simulink model "MODELofpV1MODULE"  (R2023a)
settings: Solver=VariableStepAuto  StartTime=0.0  StopTime=2  RelTol=1e-3
libraries: spsPVArrayLib x6, spsDiodeLib x3, spsControlledVoltageSourceLib x1, spsCurrentMeasurementLib x1, simulink x1, spsVoltageMeasurementLib x1, sps_lib x1
settings Model: Creator=hp  LastModifiedBy=ask
settings SolverCC: AlgebraicLoopSolver=TrustRegion
settings DataIOCC: ReturnWorkspaceOutputs=off
settings DebuggingCC: UnconnectedInputMsg=warning  UnconnectedOutputMsg=warning  UnconnectedLineMsg=warning  ArithmeticOperatorsInVariantConditions=warning
settings ModelReferenceCC: EnableRefExpFcnMdlSchedulingChecks=on
settings SFSimCC: SimUseLocalCustomCode=off  CustomCodeUndefinedFunction=UseInterfaceOnly
settings RTWCC: RTWUseLocalCustomCode=off
settings CodeAppCC: StateflowObjectComments=on
settings SimscapeCC: SimscapeNormalizeSystem=off

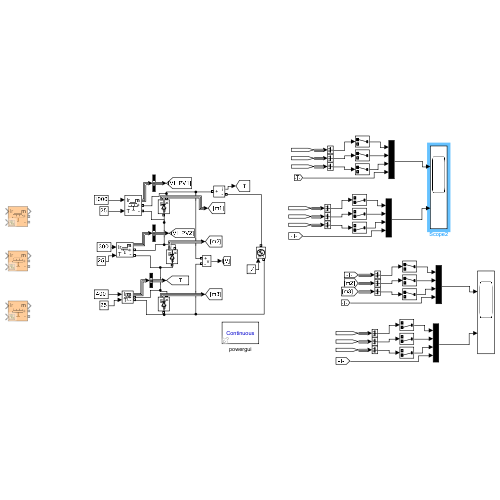
[thumbnail: Simulink's stored preview of the top-level diagram]
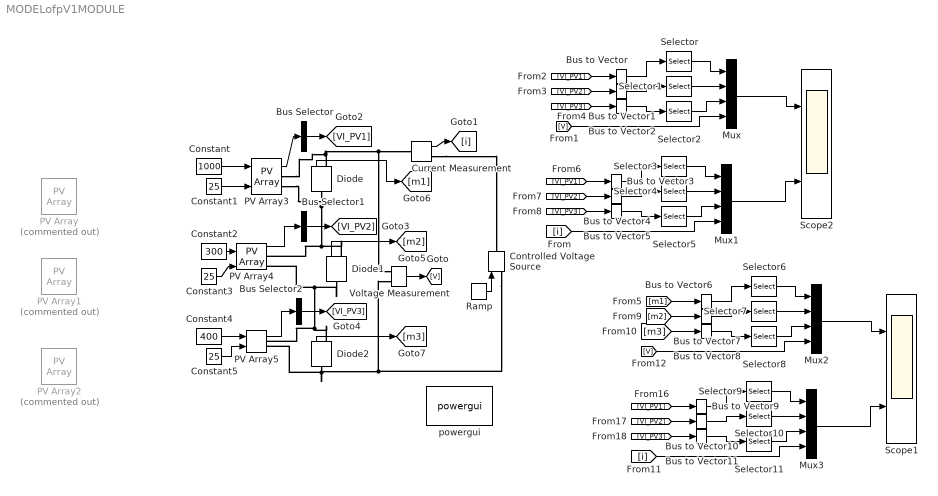
== system MODELofpV1MODULE ==
  Bus Selector : BusSelector  OutputSignals=V_PV,I_PV  OutputAsBus=on
  Bus Selector1 : BusSelector  OutputSignals=V_PV,I_PV  OutputAsBus=on
  Bus Selector2 : BusSelector  OutputSignals=V_PV,I_PV  OutputAsBus=on
  Bus to Vector{,1..11} (12 alike) : BusToVector
  Constant : Constant  Value=1000
  Constant1 : Constant  Value=25
  Constant2 : Constant  Value=300
  Constant3 : Constant  Value=25
  Constant4 : Constant  Value=400
  Constant5 : Constant  Value=25
  Controlled Voltage Source : spsControlledVoltageSourceLib/Controlled Voltage Source  Initialize=on  Source_Type=AC  Amplitude=0  Phase=0  Frequency=0  Measurements=None
  Current Measurement : spsCurrentMeasurementLib/Current Measurement  PhasorSimulation=off  OutputType=Complex  PSBequivalent=0
  Diode : spsDiodeLib/Diode  Ron=0.001  Lon=0  Vf=0.7  IC=0  UseSnubber=off  Rs=1e5*inf  Cs=inf  Measurements=on
  Diode1 : spsDiodeLib/Diode  Ron=0.001  Lon=0  Vf=0.7  IC=0  UseSnubber=off  Rs=1e5*inf  Cs=inf  Measurements=on
  Diode2 : spsDiodeLib/Diode  Ron=0.001  Lon=0  Vf=0.7  IC=0  UseSnubber=off  Rs=1e5*inf  Cs=inf  Measurements=on
  Mux{,1..3} (4 alike) : Mux
  PV Array : spsPVArrayLib/PV Array  Commented=on  Npar=1  Nser=1  PlotType=one module @ 25 deg.C & specified irradiances  S_vec="[ 1000  500  100 ]"  Temp_C_vec="[ 1000 500   ]"  ModuleName=User-defined  PlotWhenSelected=off  Pm=99.4224  Ncell=60/3  Voc=37.92*20/60  Isc=8.62  Vm=36.96*20/60  Im=8.07  beta_Voc_pc=-0.33969  alpha_Isc_pc=0.063701  beta_Voc=-0.042937  alpha_Isc=0.005491  IL=10.4557  I0=1.4325e-09  nI=1.3575  Rsh=1.8855  Rs=0.028506  RobustModel=off  RobustCellTemperature=313.3991  BAL=off  Tc=1e-6  Tfilter=5e-5
  PV Array1 : spsPVArrayLib/PV Array  Commented=on  Npar=1  Nser=1  PlotType=one module @ 25 deg.C & specified irradiances  S_vec="[ 1000  500  100 ]"  Temp_C_vec="[ 1000 500   ]"  ModuleName=User-defined  PlotWhenSelected=off  Pm=99.4224  Ncell=60/3  Voc=37.92*20/60  Isc=8.62  Vm=36.96*20/60  Im=8.07  beta_Voc_pc=-0.33969  alpha_Isc_pc=0.063701  beta_Voc=-0.042937  alpha_Isc=0.005491  IL=10.4557  I0=1.4325e-09  nI=1.3575  Rsh=1.8855  Rs=0.028506  RobustModel=off  RobustCellTemperature=313.3991  BAL=off  Tc=1e-6  Tfilter=5e-5
  PV Array2 : spsPVArrayLib/PV Array  Commented=on  Npar=1  Nser=1  PlotType=one module @ 25 deg.C & specified irradiances  S_vec="[ 1000  500  100 ]"  Temp_C_vec="[ 1000 500   ]"  ModuleName=User-defined  PlotWhenSelected=off  Pm=99.4224  Ncell=60/3  Voc=37.92*20/60  Isc=8.62  Vm=36.96*20/60  Im=8.07  beta_Voc_pc=-0.33969  alpha_Isc_pc=0.063701  beta_Voc=-0.042937  alpha_Isc=0.005491  IL=10.4557  I0=1.4325e-09  nI=1.3575  Rsh=1.8855  Rs=0.028506  RobustModel=off  RobustCellTemperature=313.3991  BAL=off  Tc=1e-6  Tfilter=5e-5
  PV Array3 : spsPVArrayLib/PV Array  Npar=1  Nser=1  PlotType=one module @ 25 deg.C & specified irradiances  S_vec="[ 1000  500  100 ]"  Temp_C_vec="[ 45 25  ]"  ModuleName=User-defined  PlotWhenSelected=off  Pm=99.4224  Ncell=60/3  Voc=37.92*20/60  Isc=8.62  Vm=36.96*20/60  Im=8.07  beta_Voc_pc=-0.36099  alpha_Isc_pc=0.063701  beta_Voc=-0.045629  alpha_Isc=0.005491  IL=10.5138  I0=5.8458e-10  nI=1.3056  Rsh=1.8742  Rs=0.043022  RobustModel=off  RobustCellTemperature=313.3991  BAL=on  Tc=1e-6  Tfilter=5e-5
  PV Array4 : spsPVArrayLib/PV Array  Npar=1  Nser=1  PlotType=one module @ 25 deg.C & specified irradiances  S_vec="[ 1000  500  100 ]"  Temp_C_vec="[ 45 25  ]"  ModuleName=User-defined  PlotWhenSelected=off  Pm=99.4224  Ncell=60/3  Voc=37.92*20/60  Isc=8.62  Vm=36.96*20/60  Im=8.07  beta_Voc_pc=-0.36099  alpha_Isc_pc=0.063701  beta_Voc=-0.045629  alpha_Isc=0.005491  IL=10.5138  I0=5.8458e-10  nI=1.3056  Rsh=1.8742  Rs=0.043022  RobustModel=off  RobustCellTemperature=313.3991  BAL=on  Tc=1e-6  Tfilter=5e-5
  PV Array5 : spsPVArrayLib/PV Array  Npar=1  Nser=1  PlotType=one module @ 25 deg.C & specified irradiances  S_vec="[ 1000  500  100 ]"  Temp_C_vec="[ 45 25  ]"  ModuleName=User-defined  PlotWhenSelected=off  Pm=99.4224  Ncell=60/3  Voc=37.92*20/60  Isc=8.62  Vm=36.96*20/60  Im=8.07  beta_Voc_pc=-0.36099  alpha_Isc_pc=0.063701  beta_Voc=-0.045629  alpha_Isc=0.005491  IL=10.5138  I0=5.8458e-10  nI=1.3056  Rsh=1.8742  Rs=0.043022  RobustModel=off  RobustCellTemperature=313.3991  BAL=on  Tc=1e-6  Tfilter=5e-5
  Ramp : simulink/Sources/Ramp  slope=37.92  start=0  InitialOutput=0
  Scope1 : Scope  NumInputPorts=2
  Scope2 : Scope  NumInputPorts=2
  Selector{,1..2,6..8} (6 alike) : Selector  InputPortWidth=2  IndexOptions=Index vector (dialog)  Indices=[1]  OutputSizes=1
  Selector{3..5,9..11} (6 alike) : Selector  InputPortWidth=2  IndexOptions=Index vector (dialog)  Indices=[2]  OutputSizes=1
  Voltage Measurement : spsVoltageMeasurementLib/Voltage Measurement  PhasorSimulation=off  OutputType=Complex  PSBequivalent=0
  powergui : sps_lib/powergui  Priority=1  SimulationMode=Continuous  SampleTime=50e-6  frequency=60  Iterations=50  frequencyindice=0  Pbase=100e6  ErrMax=1e-4  UnitsV=kV  UnitsW=MW  buscounter=0  FunctionMessages=off  echomessages=off  EnableUseOfTLC=off  CurrentSourceSwitches=off  DisableSnubberDevices=off  DisableRonSwitches=off  DisableVfSwitches=off  DisplayEquations=off  AutomaticDiscreteSolvers=off  SolverType=Tustin/Backward Euler (TBE)  Interpol=off  ExternalGateDelay=off  methode=off  Ts=10  x0status=blocks  SPID=off  SwTol=0  HookPort=off  NonlinearTolerance=1e-4  nMaxIteration=100  ContinueOnMaxIteration=off  RestoreLinks=warning  ResistiveCurrentMeasurement=off  Frange=[0:2:500]  Ylog=off  Xlog=on  ShowGrid=off  save=off  variable=ZData  structure=0  ZoomFFT=off  StartTime=0.0  cycles=1  DisplayStyle=1  fundamental=60  FreqAxis=off  MaxFrequency=1000  frequencyindicesteady=1  RmsSteady=1  display=off
  wires:
  Constant/1 -> PV Array3/1
  Constant1/1 -> PV Array3/2
  Constant2/1 -> PV Array4/1
  Constant3/1 -> PV Array4/2
  Constant4/1 -> PV Array5/1
  Constant5/1 -> PV Array5/2
  PV Array3/1 -> Bus Selector/1
  PV Array4/1 -> Bus Selector1/1
  PV Array5/1 -> Bus Selector2/1
  Voltage Measurement/1 -> [V]
  Current Measurement/1 -> [i]
  Ramp/1 -> Controlled Voltage Source/1
  Bus Selector/1 -> [VI_PV1]
  Bus Selector1/1 -> [VI_PV2]
  Bus Selector2/1 -> [VI_PV3]
  Selector/1 -> Mux/1
  Selector1/1 -> Mux/2
  Selector2/1 -> Mux/3
  [V] -> Mux/4
  [VI_PV1] -> Bus to Vector/1
  [VI_PV2] -> Bus to Vector1/1
  [VI_PV3] -> Bus to Vector2/1
  Bus to Vector/1 -> Selector/1
  Bus to Vector1/1 -> Selector1/1
  Bus to Vector2/1 -> Selector2/1
  Selector3/1 -> Mux1/1
  Selector4/1 -> Mux1/2
  Selector5/1 -> Mux1/3
  [i] -> Mux1/4
  [VI_PV1] -> Bus to Vector3/1
  [VI_PV2] -> Bus to Vector4/1
  [VI_PV3] -> Bus to Vector5/1
  Bus to Vector3/1 -> Selector3/1
  Bus to Vector4/1 -> Selector4/1
  Bus to Vector5/1 -> Selector5/1
  Mux/1 -> Scope2/1
  Mux1/1 -> Scope2/2
  Diode1/1 -> [m2]
  Diode/1 -> [m1]
  Diode2/1 -> [m3]
  Selector6/1 -> Mux2/1
  Selector7/1 -> Mux2/2
  Selector8/1 -> Mux2/3
  [V] -> Mux2/4
  [m1] -> Bus to Vector6/1
  [m2] -> Bus to Vector7/1
  [m3] -> Bus to Vector8/1
  Bus to Vector6/1 -> Selector6/1
  Bus to Vector7/1 -> Selector7/1
  Bus to Vector8/1 -> Selector8/1
  Selector9/1 -> Mux3/1
  Selector10/1 -> Mux3/2
  Selector11/1 -> Mux3/3
  [i] -> Mux3/4
  [VI_PV1] -> Bus to Vector9/1
  [VI_PV2] -> Bus to Vector10/1
  [VI_PV3] -> Bus to Vector11/1
  Bus to Vector9/1 -> Selector9/1
  Bus to Vector10/1 -> Selector10/1
  Bus to Vector11/1 -> Selector11/1
  Mux2/1 -> Scope1/1
  Mux3/1 -> Scope1/2
  connections:
  Diode/RConn1 -- PV Array3/RConn1 -- Voltage Measurement/LConn1 -- Current Measurement/LConn1
  Diode/LConn1 -- PV Array3/RConn2 -- PV Array4/RConn1 -- Diode1/RConn1
  Diode1/LConn1 -- PV Array4/RConn2 -- PV Array5/RConn1 -- Diode2/RConn1
  Diode2/LConn1 -- PV Array5/RConn2 -- Controlled Voltage Source/LConn1 -- Voltage Measurement/LConn2
  Current Measurement/RConn1 -- Controlled Voltage Source/RConn1
